simulink model "pick_rotate"  (R2019a)
settings: Solver=FixedStepAuto  StartTime=0.0  StopTime=t_sim  RelTol=1e-3
values from neighbouring files (symbols this model uses):
  adap_init =     [matlab.mat]
  den =     [matlab.mat]
  F = 1.9    [matlab.mat]    (also in model_update.m = Tau; pick.m = Tau)
  Gpm = [0.9 0.1 ... (first row only)    [pick.m]
  Init_ck = [0.9 0.1]    [pick.m]
  noise_gain = 0    [matlab.mat]    (also in pick.m)
  num =     [matlab.mat]
  t_AdapOff = 5    [matlab.mat]    (also in pick.m)
  t_AdapOn = 0    [matlab.mat]    (also in pick.m)
  Ts = 0.01    [matlab.mat]    (also in pick.m)
libraries: simulink x4
settings Model: Creator=litingsun  LastModifiedBy=jessl
settings DataIOCC: ReturnWorkspaceOutputs=off
settings DebuggingCC: ArithmeticOperatorsInVariantConditions=warning
settings SFSimCC: SimUseLocalCustomCode=off
settings RTWCC: RTWUseLocalCustomCode=off
settings CodeAppCC: StateflowObjectComments=on

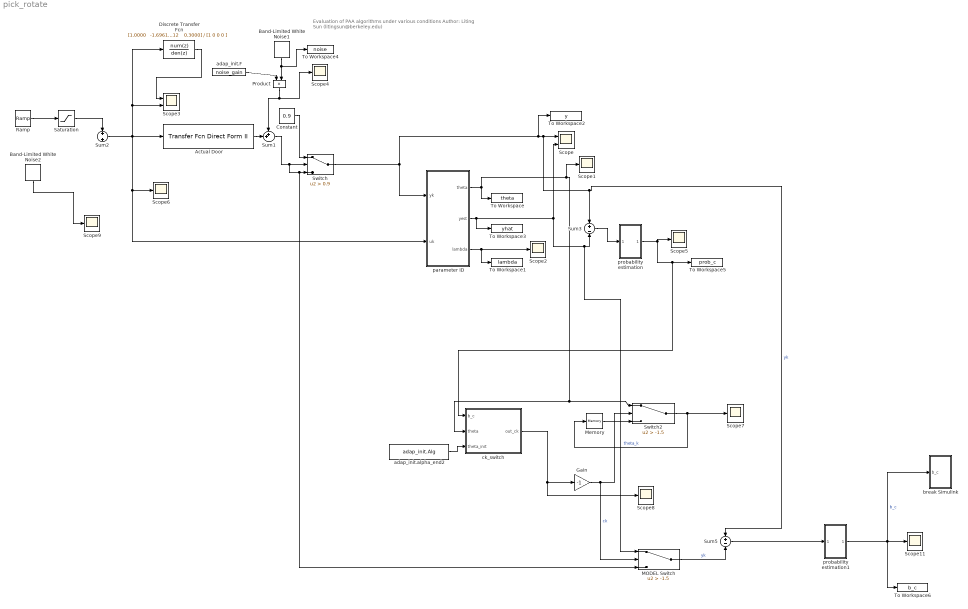
== system pick_rotate ==
  note: Evaluation of PAA algorithms under various conditions
      |
      | Author: Liting Sun (litingsun@berkeley.edu)
  Actual Door : simulink/Additional Math & Discrete/Additional Discrete/Transfer Fcn Direct Form II  NumCoefVec=num{1}  DenCoefVec=den{1}(2:3)  vinit=0.0  RndMeth=Zero  DoSatur=off
      settings: SourceProductName=Simulink  SourceProductBaseCode=SL
  Band-Limited White Noise1 : simulink/Sources/Band-Limited White Noise  Cov=[1]  Ts=Ts  seed=[12345]
  Band-Limited White Noise2 : simulink/Sources/Band-Limited White Noise  Cov=[0.1]  Ts=Ts  seed=[12345]
  Constant : Constant  Value=0.9
  Discrete Transfer Fcn : DiscreteTransferFcn  Numerator="[1.0000   -1.6961    0.4012    0.3000]"  Denominator=[1 0 0 0 ]
  Gain : Gain  Gain=-1
  MODEL Switch : Switch  Criteria=u2 > Threshold  Threshold=-1.5
  Memory : Memory
  Product : Product
  Ramp : simulink/Sources/Ramp  slope=2  start=0.5  InitialOutput=0
  Saturation : Saturate  UpperLimit=F
  Scope : Scope  NumInputPorts=2
  Scope{1..2,4..9,11} (9 alike) : Scope
  Scope3 : Scope  NumInputPorts=2
  Sum1 : Sum  Inputs=++|
  Sum2 : Sum  Inputs=+||+
  Sum3 : Sum  Inputs=+-
  Sum5 : Sum  Inputs=+-
  Switch : Switch  Criteria=u2 > Threshold  Threshold=0.9
  Switch2 : Switch  Criteria=u2 > Threshold  Threshold=-1.5
  To Workspace : ToWorkspace  VariableName=theta  SaveFormat=Structure With Time  SampleTime=-1
  To Workspace1 : ToWorkspace  VariableName=lambda  SaveFormat=Structure With Time  SampleTime=-1
  To Workspace2 : ToWorkspace  VariableName=y  SaveFormat=Structure With Time  SampleTime=-1
  To Workspace3 : ToWorkspace  VariableName=yhat  SaveFormat=Structure With Time  SampleTime=-1
  To Workspace4 : ToWorkspace  VariableName=noise  SaveFormat=Structure With Time  SampleTime=-1
  To Workspace5 : ToWorkspace  VariableName=prob_c  SaveFormat=Structure With Time  SampleTime=-1
  To Workspace6 : ToWorkspace  VariableName=b_c  SaveFormat=Structure With Time  SampleTime=-1
  "adap_init.F " : Constant  Value=noise_gain
  adap_init.alpha_end2 : Constant  Value=adap_init.Alg
  break Simulink : Subsystem
  ck_switch : MATLAB Function  TreatAsAtomicUnit=on
  parameter ID : Subsystem
  probability estimation : Subsystem
  probability estimation1 : Subsystem
  wires:
  parameter ID/3(lambda) -> Scope2/1, To Workspace1/1
  parameter ID/2(yest) -> MODEL Switch/1, Sum3/2, Scope/2, To Workspace3/1
  Actual Door/1 -> Sum1/2
  Band-Limited White Noise1/1 -> To Workspace4/1, Product/2
  Product/1 -> Scope4/1, Sum1/1
  "adap_init.F "/1 -> Product/1
  Sum1/1 -> MODEL Switch/3, Switch/3, Switch/2
  Discrete Transfer Fcn/1 -> Scope3/1
  Switch/1 -> parameter ID/1(yk), Sum5/1, Sum3/1, Scope/1, To Workspace2/1  "yk"
  parameter ID/1(theta) -> ck_switch/2(theta), Switch2/1, Scope1/1, To Workspace/1
  Sum3/1 -> probability estimation/1(In1)
  Constant/1 -> Switch/1
  Switch2/1 -> Memory/1, Scope7/1  "theta_k"
  Memory/1 -> Switch2/3
  adap_init.alpha_end2/1 -> ck_switch/3(theta_init)
  ck_switch/1(out_ck) -> Gain/1, Scope8/1
  Gain/1 -> MODEL Switch/2, Switch2/2  "ck"
  MODEL Switch/1 -> Sum5/2  "yk"
  Saturation/1 -> Sum2/1
  Sum5/1 -> probability estimation1/1(In1)
  probability estimation/1(Out1) -> Scope5/1, ck_switch/1(b_c), To Workspace5/1
  probability estimation1/1(Out1) -> break Simulink/1(b_c), To Workspace6/1, Scope11/1  "b_c"
  Ramp/1 -> Saturation/1
  Band-Limited White Noise2/1 -> Scope9/1
  Sum2/1 -> Scope6/1, parameter ID/2(uk), Actual Door/1, Scope3/2, Discrete Transfer Fcn/1

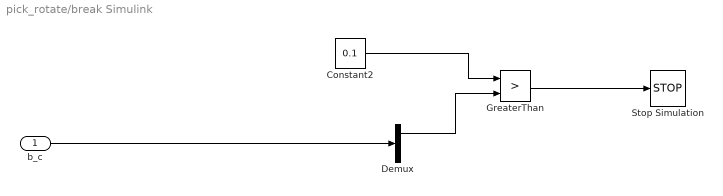
== system pick_rotate/break Simulink ==
  b_c : Inport
  Constant2 : Constant  Value=0.1
  Demux : Demux  Outputs=2
  GreaterThan : RelationalOperator  Operator=>  OutDataTypeStr=boolean  RndMeth=Simplest
  Stop Simulation : Stop
  wires:
  GreaterThan/1 -> Stop Simulation/1
  Constant2/1 -> GreaterThan/1
  b_c/1 -> Demux/1
  Demux/1 -> GreaterThan/2

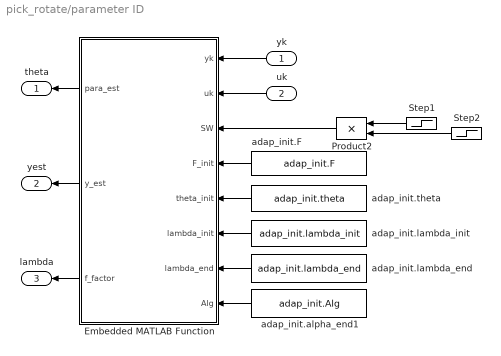
== system pick_rotate/parameter ID ==
  yk : Inport
  uk : Inport  Port=2
  Embedded MATLAB Function : MATLAB Function  TreatAsAtomicUnit=on
  Product2 : Product  RndMeth=Zero
  Step1 : Step  Time=t_AdapOn  SampleTime=Ts
  Step2 : Step  Time=t_AdapOff  Before=1  After=0  SampleTime=Ts
  "adap_init.F " : Constant  Value=adap_init.F
  adap_init.alpha_end1 : Constant  Value=adap_init.Alg
  adap_init.lambda_end : Constant  Value=adap_init.lambda_end
  adap_init.lambda_init : Constant  Value=adap_init.lambda_init
  adap_init.theta : Constant  Value=adap_init.theta
  theta : Outport
  yest : Outport  Port=2
  lambda : Outport  Port=3
  wires:
  uk/1 -> Embedded MATLAB Function/2(uk)
  Embedded MATLAB Function/3(f_factor) -> lambda/1
  "adap_init.F "/1 -> Embedded MATLAB Function/4(F_init)
  adap_init.alpha_end1/1 -> Embedded MATLAB Function/8(Alg)
  Embedded MATLAB Function/1(para_est) -> theta/1
  adap_init.lambda_init/1 -> Embedded MATLAB Function/6(lambda_init)
  yk/1 -> Embedded MATLAB Function/1(yk)
  adap_init.lambda_end/1 -> Embedded MATLAB Function/7(lambda_end)
  Product2/1 -> Embedded MATLAB Function/3(SW)
  Step2/1 -> Product2/2
  Step1/1 -> Product2/1
  adap_init.theta/1 -> Embedded MATLAB Function/5(theta_init)
  Embedded MATLAB Function/2(y_est) -> yest/1

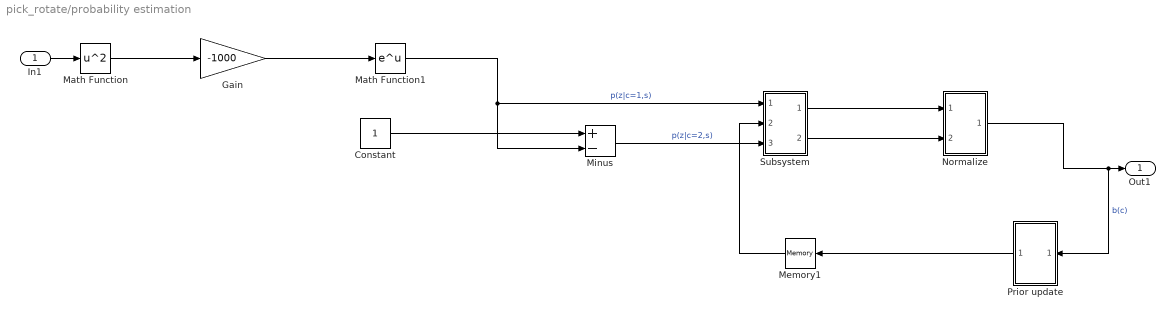
== system pick_rotate/probability estimation ==
  In1 : Inport
  Constant : Constant
  Gain : Gain  Gain=-1000
  Math Function : Math  Operator=square  SaturateOnIntegerOverflow=on
  Math Function1 : Math  SaturateOnIntegerOverflow=on
  Memory1 : Memory  InitialCondition=Init_ck
  Minus : Sum  Inputs=+-
  Normalize : Subsystem
  Prior update : Subsystem
  Subsystem : Subsystem
  Out1 : Outport
  wires:
  Gain/1 -> Math Function1/1
  Math Function/1 -> Gain/1
  In1/1 -> Math Function/1
  Constant/1 -> Minus/1
  Normalize/1(Out1) -> Prior update/1(In1), Out1/1  "b(c)"
  Prior update/1(Out1) -> Memory1/1
  Math Function1/1 -> Subsystem/1(In1), Minus/2  "p(z|c=1,s)"
  Memory1/1 -> Subsystem/2(In2)
  Minus/1 -> Subsystem/3(In3)  "p(z|c=2,s)"
  Subsystem/1(Out1) -> Normalize/1(In1)
  Subsystem/2(Out2) -> Normalize/2(In2)

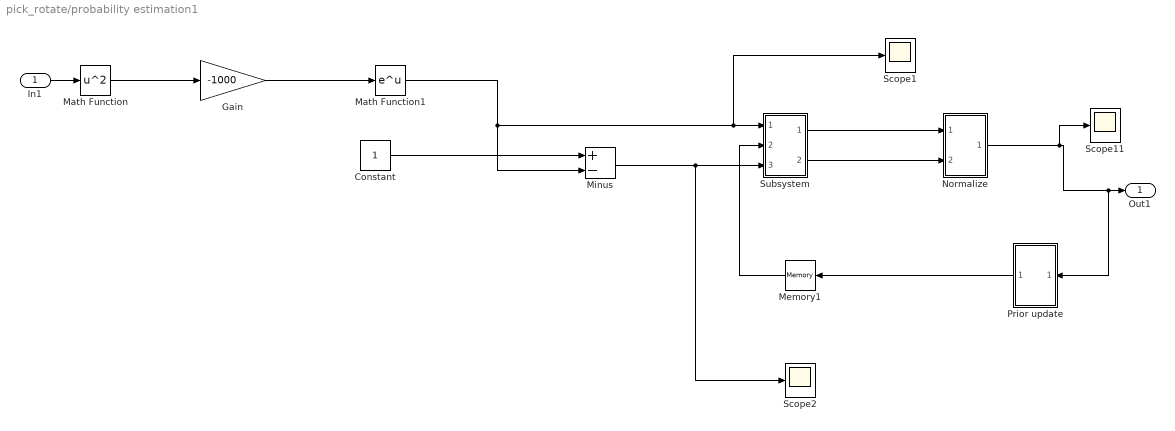
== system pick_rotate/probability estimation1 ==
  In1 : Inport
  Constant : Constant
  Gain : Gain  Gain=-1000
  Math Function : Math  Operator=square  SaturateOnIntegerOverflow=on
  Math Function1 : Math  SaturateOnIntegerOverflow=on
  Memory1 : Memory  InitialCondition=Init_ck
  Minus : Sum  Inputs=+-
  Normalize : Subsystem
  Prior update : Subsystem
  Scope1 : Scope
  Scope11 : Scope
  Scope2 : Scope
  Subsystem : Subsystem
  Out1 : Outport
  wires:
  Gain/1 -> Math Function1/1
  Math Function/1 -> Gain/1
  In1/1 -> Math Function/1
  Constant/1 -> Minus/1
  Normalize/1(Out1) -> Scope11/1, Prior update/1(In1), Out1/1
  Prior update/1(Out1) -> Memory1/1
  Math Function1/1 -> Scope1/1, Subsystem/1(In1), Minus/2
  Memory1/1 -> Subsystem/2(In2)
  Minus/1 -> Scope2/1, Subsystem/3(In3)
  Subsystem/1(Out1) -> Normalize/1(In1)
  Subsystem/2(Out2) -> Normalize/2(In2)

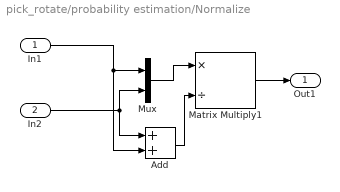
== system pick_rotate/probability estimation/Normalize ==
  In1 : Inport
  In2 : Inport  Port=2
  Add : Sum
  Matrix Multiply1 : Product  Inputs=*/
  Mux : Mux  Inputs=2
  Out1 : Outport
  wires:
  In2/1 -> Mux/2, Add/1
  Add/1 -> Matrix Multiply1/2
  In1/1 -> Add/2, Mux/1
  Mux/1 -> Matrix Multiply1/1
  Matrix Multiply1/1 -> Out1/1

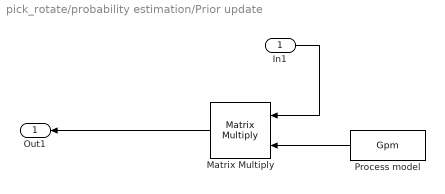
== system pick_rotate/probability estimation/Prior update ==
  In1 : Inport
  Matrix Multiply : Product  Multiplication=Matrix(*)
  Process model : Constant  Value=Gpm  VectorParams1D=off
  Out1 : Outport
  wires:
  Process model/1 -> Matrix Multiply/2
  In1/1 -> Matrix Multiply/1
  Matrix Multiply/1 -> Out1/1

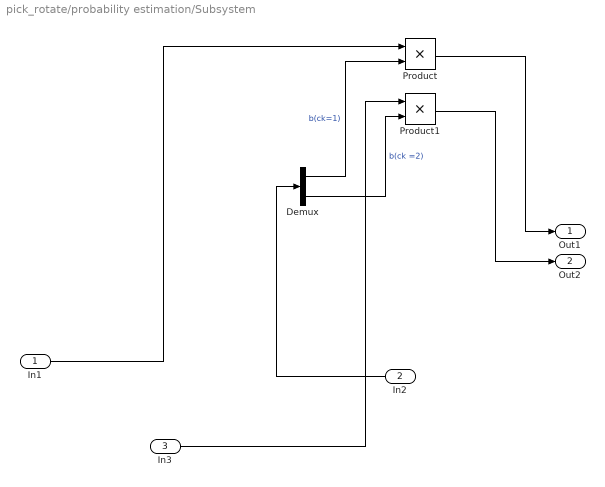
== system pick_rotate/probability estimation/Subsystem ==
  In1 : Inport
  In2 : Inport  Port=2
  In3 : Inport  Port=3
  Demux : Demux  Outputs=2
  Product : Product
  Product1 : Product
  Out1 : Outport
  Out2 : Outport  Port=2
  wires:
  In3/1 -> Product1/1
  Product/1 -> Out1/1
  Demux/1 -> Product/2  "b(ck=1)"
  Product1/1 -> Out2/1
  Demux/2 -> Product1/2  "b(ck =2)"
  In2/1 -> Demux/1
  In1/1 -> Product/1

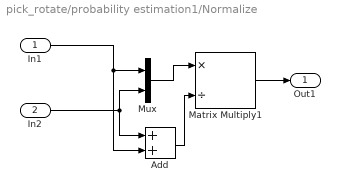
== system pick_rotate/probability estimation1/Normalize ==
  In1 : Inport
  In2 : Inport  Port=2
  Add : Sum
  Matrix Multiply1 : Product  Inputs=*/
  Mux : Mux  Inputs=2
  Out1 : Outport
  wires:
  In2/1 -> Mux/2, Add/1
  Add/1 -> Matrix Multiply1/2
  In1/1 -> Add/2, Mux/1
  Mux/1 -> Matrix Multiply1/1
  Matrix Multiply1/1 -> Out1/1

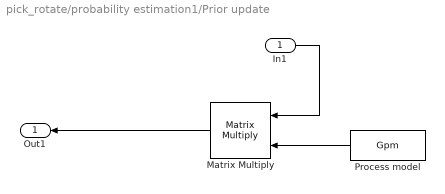
== system pick_rotate/probability estimation1/Prior update ==
  In1 : Inport
  Matrix Multiply : Product  Multiplication=Matrix(*)
  Process model : Constant  Value=Gpm  VectorParams1D=off
  Out1 : Outport
  wires:
  Process model/1 -> Matrix Multiply/2
  In1/1 -> Matrix Multiply/1
  Matrix Multiply/1 -> Out1/1

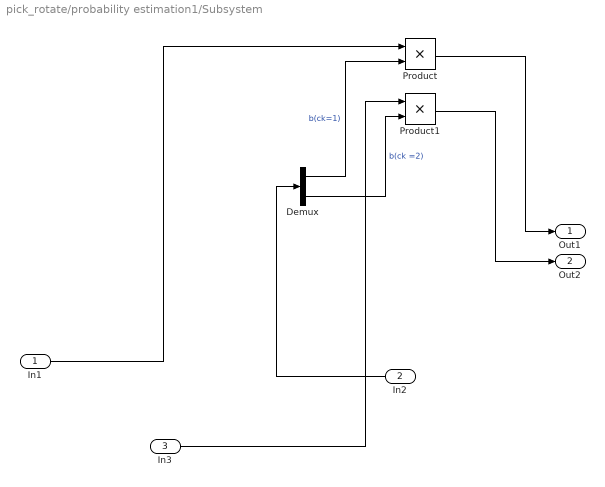
== system pick_rotate/probability estimation1/Subsystem ==
  In1 : Inport
  In2 : Inport  Port=2
  In3 : Inport  Port=3
  Demux : Demux  Outputs=2
  Product : Product
  Product1 : Product
  Out1 : Outport
  Out2 : Outport  Port=2
  wires:
  In3/1 -> Product1/1
  Product/1 -> Out1/1
  Demux/1 -> Product/2  "b(ck=1)"
  Product1/1 -> Out2/1
  Demux/2 -> Product1/2  "b(ck =2)"
  In2/1 -> Demux/1
  In1/1 -> Product/1

== matlab function pick_rotate/ck_switch ==
  data: out_ck output; b_c input; theta input; theta_init input
function out_ck  = ck_switch(b_c,theta,theta_init) 

persistent N ck stor_th
if isempty(N)
    % initialize all necessary parameters     
    N       = uint16(1);
    ck      = 1; 
    stor_th = theta_init;
end

switch(ck)
    case 1
        if b_c[1]<0.7
            ck = 2;
            
        end
        
        if b_c[1]>0.7 
            stor_th = theta;
        end
        
        
    case 2
        if b_c[1]>0.95
            stor_th = theta;
        end
        if b_c[1]<0.5
            %ck = 1;
        end
end
        
out_ck = ck;
%out_theta = stor_th;

== matlab function pick_rotate/parameter ID/Embedded MATLAB Function ==
  data: yk input; uk input; SW input; para_est output; y_est output; f_factor output; F_init input; theta_init input; lambda_init input; lambda_end input; Alg input
function [para_est, y_est, f_factor] = PAA(yk,uk, SW, F_init,theta_init,lambda_init,lambda_end, Alg) %#eml
persistent N y u phi F theta lambda yhat ehat ykhat ek vk iter phi_F_phi delta_theta;
persistent ykhat_post ek_post flag_series_parallel theta_comp; 
% PAA algorithms implementation for two order systems: 
% two numberator parameters and two denominator parameters
%                 b0+b1*z^-1
% y(k) = ----------------------u(k-1)
%            1+a1*z^-1 +a2*z^-2
% ==> theta = [a1, a2, b0, b1]', phi = [-y(k-1), -y(k-2), u(k-1), u(k-2)]';
% ============================================================
%   Copyright (c) 2015-, Liting Sun, litingsun@berkeley.edu
%   Author(s): Liting Sun
%              University of California at Berkeley
%              Berkeley, CA, 94720, USA
% ============================================================
if isempty(N)
    % initialize all necessary parameters     
    N       = uint16(1);
    y       = zeros(2,1);
    yhat    = zeros(2,1);
    ehat    = zeros(2,1); % store the posterior estimation error
    u       = zeros(2,1);
    phi     = zeros(4,1);
    
    F       = F_init;
    theta   = theta_init; 
    lambda  = lambda_init;
    
    ykhat       = 0;
    ykhat_post  = 0;
    ek          = 0;
    ek_post     = 0;
    
    iter        = 0;
    phi_F_phi   = 0;
    delta_theta = 0*theta_init;
    
    flag_series_parallel = 1;
    theta_comp  = theta;
    
end
if SW == 0
    %========= Adaptation turned off. ==========
    % update observation vector
    ykhat     = [-yhat(1), -yhat(2), u(1), u(2)]*theta;
    
    y(2)     = y(1);
    y(1)     = yk;
    u(2)     = u(1);
    u(1)     = uk;
    yhat(2)  = yhat(1);
    yhat(1)  = yk;
    
    para_est = theta;
    f_factor = lambda;
    y_est    = ykhat;
    
    
else
    switch(Alg)
        case 0 % series-parallel structure
            %% read data
            phi = [-y(1), -y(2), u(1), u(2)]';
            % a priori estimate
            ykhat = phi'*theta;
            % a priori estimation error
            ek = yk - ykhat;
            phi_F_phi = phi'*F*phi;
            delta_theta = (F*phi*ek/(1+phi_F_phi));
            % parameter estimation update
            theta = theta + delta_theta;
            % adaptation gain update
            F = 1/lambda * ( F - F*(phi*phi')*F / (lambda+phi_F_phi) );
            % a posteriori prediction
            ykhat_post = phi'*theta;
            ek_post = yk - ykhat_post;
            % update the forgetting factor
            lambda = lambda_end - (lambda_end-lambda) * 0.98;
            % update observation vector
            y(2)     = y(1);
            y(1)     = yk;
            u(2)     = u(1);
            u(1)     = uk;
            
        case 1     % parallel structure
            %% read data
            phi = [-yhat(1), -yhat(2), u(1), u(2)]';
            % a priori estimation 
            ykhat = phi'*theta;
            % a priori estimation error
            ek = yk - ykhat;
            phi_F_phi = phi'*F*phi;
            % parameter estimation update
            delta_theta = (F*phi*ek/(1+phi_F_phi));
            theta = theta + delta_theta;
            F = 1/lambda * ( F - F*(phi*phi')*F / (lambda+phi_F_phi) );
            % a posteriori prediction
            ykhat_post = phi'*theta;
            ek_post = yk - ykhat_post;
            lambda = lambda_end - (lambda_end-lambda) * 0.98;
            % update observation vector
            u(2)     = u(1);
            u(1)     = uk;
            yhat(2) = yhat(1);
            yhat(1) = ykhat_post;
        case 2      
            % parallel structure with a fixed compensator and the fixed compensator comes from sp-PAA
            % i.e, we are using two-stage PAA
            %% first stage: sp PAA for a rough estimation
            if flag_series_parallel == 1
                % read data
                phi = [-y(1), -y(2), u(1), u(2)]';
                % a priori estimate
                ykhat = phi'*theta;
                % a priori estimation error
                ek = yk - ykhat;
                phi_F_phi = phi'*F*phi;
                delta_theta = (F*phi*ek/(1+phi_F_phi));
                % parameter estimation update
                theta = theta + delta_theta;
                % adaptation gain update
                F = 1/lambda * ( F - F*(phi*phi')*F / (lambda+phi_F_phi) );
                % a posteriori prediction
                ykhat_post = phi'*theta;
                ek_post = yk - ykhat_post;
                % update the forgetting factor
                lambda = lambda_end - (lambda_end-lambda) * 0.98;
                % update observation vector
                y(2)     = y(1);
                y(1)     = yk;
                u(2)     = u(1);
                u(1)     = uk;
                yhat(2)  = yhat(1);
                yhat(1)  = yk;
                ehat(2)  = ehat(1);
                ehat(1)  = ek_post;
                if iter >= 300 % terminate the sp PAA after a fixed number of iterations
                    % set the flag to zero
                    flag_series_parallel = 0;
                    % reset the adaptation gain. It does not necessarily be
                    % F_init, and you are free to set it other values. The
                    % goal here is to make the adaptation gain large enough
                    % so that the second stage is effective.
                    F = F_init;
                    % set the current theta as the compensator coefficients
                    theta_comp = theta;
                end
            else
                % read data
                phi = [-yhat(1), -yhat(2), u(1), u(2)]';
                % a priori estimation 
                ykhat = phi'*theta;
                % a priori estimation error
                ek = yk - ykhat;
                phi_F_phi = phi'*F*phi;
                vk = ek + theta_comp(1)*ehat(1)+theta_comp(2)*ehat(2);
                % parameter estimation update
                delta_theta = (F*phi*vk/(1+phi_F_phi));
                theta = theta + delta_theta;
                F = 1/lambda * ( F - F*(phi*phi')*F / (lambda+phi_F_phi) );
                % a posteriori prediction
                ykhat_post = phi'*theta;
                ek_post = yk - ykhat_post;
                lambda = lambda_end - (lambda_end-lambda) * 0.98;
                % update observation vector
                u(2)     = u(1);
                u(1)     = uk;
                yhat(2) = yhat(1);
                yhat(1) = ykhat_post;
                ehat(2)  = ehat(1);
                ehat(1)  = ek_post;
            end
            
    end
    
    iter = iter + 1; % iteration update
    % +++++++++++++++++++++++++++++++++++++++++++
    para_est = theta;
    f_factor = lambda;
    y_est    = ykhat_post;
end
